simulink model "obiekt2"  (R2016b)
settings: Solver=VariableStepAuto  StartTime=0.0  StopTime=10.0  RelTol=1e-3
undefined symbols (not defined in the file or in its folder): A, B
settings Model: Creator=kamil  LastModifiedBy=kamil

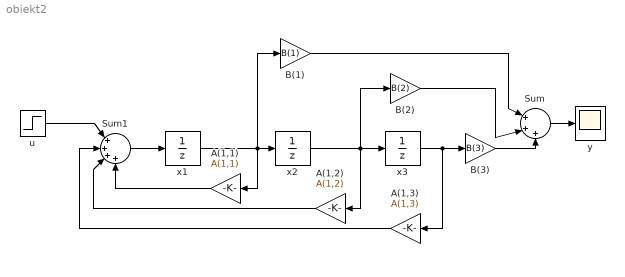
== system obiekt2 ==
  A(1,1) : Gain  Gain=A(1,1)
  A(1,2) : Gain  Gain=A(1,2)
  A(1,3) : Gain  Gain=A(1,3)
  B(1) : Gain  Gain=B(1)
  B(2) : Gain  Gain=B(2)
  B(3) : Gain  Gain=B(3)
  Sum : Sum  Inputs=|+++
  Sum1 : Sum  Inputs=|++++
  u : Step  After=0.1  SampleTime=0
  "x1 " : UnitDelay  SampleTime=-1
  x2 : UnitDelay  SampleTime=-1
  x3 : UnitDelay  SampleTime=-1
  y : Scope
  wires:
  Sum/1 -> y/1
  u/1 -> Sum1/1
  x2/1 -> B(2)/1, A(1,2)/1, x3/1
  Sum1/1 -> "x1 "/1
  x3/1 -> B(3)/1, A(1,3)/1
  A(1,3)/1 -> Sum1/2
  A(1,2)/1 -> Sum1/3
  A(1,1)/1 -> Sum1/4
  B(3)/1 -> Sum/3
  "x1 "/1 -> B(1)/1, A(1,1)/1, x2/1
  B(2)/1 -> Sum/2
  B(1)/1 -> Sum/1
